simulink model "log_map_tl"  (Simulink 6.4)
settings: Solver=FixedStepDiscrete  StartTime=0.0  StopTime=50.0  FixedStep=0.1  RelTol=1e-3
PreLoadFcn:
  | if exist('tl_preloadfcn','file'), tl_preloadfcn(gcs,95); end
PostLoadFcn:
  | if exist('tl_postloadfcn','file'), tl_postloadfcn(gcs,95); end
InitFcn:
  | if exist('tlds_start','file'), tlds_start(gcs); end
undefined symbols (not defined in the file or in its folder): built, constant, Constant, Gain, in, lambda, Product, Saturate, Sum, UnitDelay, y1_0, y2_0
libraries: tllib x33
PreSaveFcn:
  | if exist('tl_presavefcn','file'), tl_presavefcn(gcs); end
settings Model: LastModifiedBy=alexh  DS_PROJECTFILE=log_map_tl.dd  TL_MAIN_DATA=struct('maxnumsimulations',10,'codeopt',struct('inliningthreshold',6,'target',['Generic ANSI-C'],'assembler',0,'optlevel',2,'linebreaklimit',100,'stateactcodinglimit',5,'functionsfor64bitops',1,'sections',1,'sfbitfields',1,'globalbitfields',0,'sharefunctions',0,'noinitstozero',0,'limidentlength',1,'decimals',1,'separatesearch',0,'cleancode',0,'optimizedbooltype',1,'keepsaturation',0,'extvarsharing',0,'outputstylefile','cconfig.xml','rootstylesheet','TL_CSourceCodeSS.xsl','addchecksum',0,'modelsaving',2,'browsecodegen',0),'frameopt',struct('exectime',1,'stacksize',1,'simconfig',['default EVM'],'targettimeout',1,'mexargs','','tcargs',''),'logopt',struct('plotinterval',0.1,'globalloggingmode',1),'export',struct('directory','.\export','sysfiles',1,'docfiles',0,'tools',0),'asapscript','asap2_all_in_one','docscript','tldoc_default','date',733152.55044912035,'codecoveragelevel',0,'rtos',struct('enablemultirate',0,'currentrtos',['generic RTOS'],'autopriority',0,'autoinitalarm',1,'alarminitwithrestart',1,'alarmactivationkind',1,'alarmstartoffset',0))  TL_MODEL_COMMENT=Type in your documentation HERE
settings DataIOCC: LimitDataPoints=off  SaveOutput=off  SaveTime=off
settings OptimizationCC: BooleanDataType=off
settings DebuggingCC: SolverPrmCheckMsg=none  StrictBusMsg=None
settings HardwareCC: TargetUnknown=on
settings GRTTargetCC: ModelReferenceCompliant=off  MatFileLogging=off

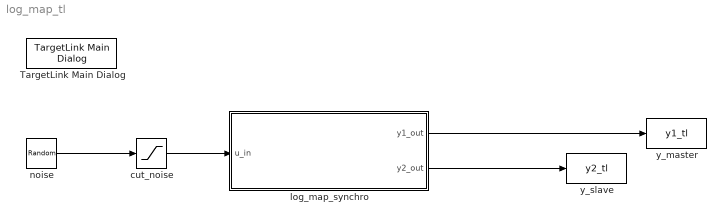
== system log_map_tl ==
  TargetLink Main Dialog : tllib/TargetLink Main Dialog  SystemSampleTime=-1  flp_block=none
  cut_noise : Saturate  UpperLimit=1  LowerLimit=0
  log_map_synchro : Subsystem  Tag=TargetLink Simulation Frame
      settings: CopyFcn=if exist('tl_copyfcn','file'), tl_copyfcn(gcbh); end  NameChangeFcn=if exist('tl_framenamechangefcn','file'), tl_framenamechangefcn(gcbh); end  OpenFcn=if exist('open_tlsubsystem','file'), open_tlsubsystem(gcbh); end
      mask Type: TL_SimFrame
      mask Display: disp('TargetLink\nModel-\nin-the-loop\nmode')
  noise : RandomNumber  Mean=0.5  SampleTime=0
  y_master : ToWorkspace  VariableName=y1_tl  SampleTime=-1  SaveFormat=Array
  y_slave : ToWorkspace  VariableName=y2_tl  SampleTime=-1  SaveFormat=Array
  wires:
  noise/1 -> cut_noise/1
  log_map_synchro/1(y1_out) -> y_master/1
  cut_noise/1 -> log_map_synchro/1(u_in)
  log_map_synchro/2(y2_out) -> y_slave/1

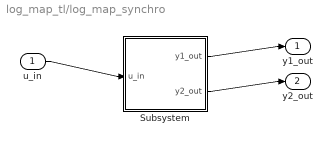
== system log_map_tl/log_map_synchro ==
  u_in : Inport  PortDimensions=1  SampleTime=0.1
      settings: NameChangeFcn=tl_check_ports(gcbh);
  Subsystem : Subsystem  Tag=struct('sfcnName','log_map_synchro_sf','subFunction','','srcSubsystem','')
      settings: OpenFcn=warndlg(get_param(gcb,'MaskHelp'),'Serious Warning');
      mask Type: TL_Enable
      mask Help: This subsystem keeps the TargetLink subsystem (subsystem with TargetLink blocks for production code generation), and is needed for the TargetLink simulation frame to work properly. DO NOT DELETE OR MODIFY IT!
  y1_out : Outport
  y2_out : Outport  Port=2
      settings: NameChangeFcn=tl_check_ports(gcbh);
  wires:
  u_in/1 -> Subsystem/1(u_in)
  Subsystem/1(y1_out) -> y1_out/1
  Subsystem/2(y2_out) -> y2_out/1

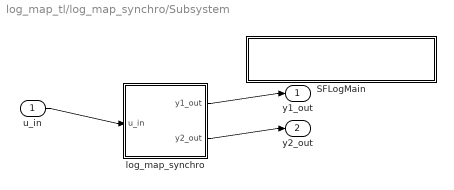
== system log_map_tl/log_map_synchro/Subsystem ==
  u_in : Inport  PortDimensions=1  SampleTime=0.1
      settings: NameChangeFcn=tl_check_ports(gcbh);
  SFLogMain : Subsystem
      mask Type: TL_StateflowLoggingMain
      mask Display:
      | plot([0 0 1 1 0 0 1 1 0],[0 1 1 0 0 0.05 0.05 0.95 0.95]);
      | disp('Stateflow Logging Main\nDO NOT DELETE')
  log_map_synchro : Subsystem  Tag=MIL Subsystem  Description=b
      settings: CopyFcn=if exist('tl_copyfcn','file'), tl_copyfcn(gcbh); end  NameChangeFcn=if exist('tl_namechangefcn','file'), tl_namechangefcn(gcbh); end  DestroyFcn=if exist('update_tl_main_dlg','file'), update_tl_main_dlg('TL_subs_display'); end
  y1_out : Outport
  y2_out : Outport  Port=2
      settings: NameChangeFcn=tl_check_ports(gcbh);
  wires:
  u_in/1 -> log_map_synchro/1(u_in)
  log_map_synchro/1(y1_out) -> y1_out/1
  log_map_synchro/2(y2_out) -> y2_out/1

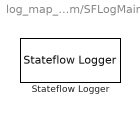
== system log_map_tl/log_map_synchro/Subsystem/SFLogMain ==
  Stateflow Logger : tllib/Extras/Stateflow Logger  data=struct('date',730486)  sflogparam=struct('charts',[],'sfblocks',[],'machines',[],'globallogopt',1,'modelname','log_map_tl','debugmodeactive',0)  flp_block=tldummylib/Stateflow Logger

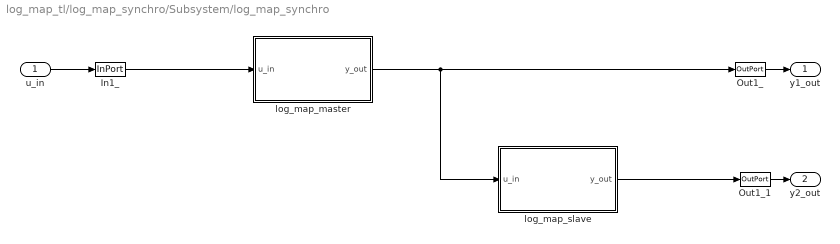
== system log_map_tl/log_map_synchro/Subsystem/log_map_synchro ==
  u_in : Inport  PortDimensions=1  SampleTime=0.1
      settings: CopyFcn=if exist('tl_check_ports','file'), tl_check_ports(gcbh); end  NameChangeFcn=if exist('tl_check_ports','file'), tl_check_ports(gcbh); end
  In1_ : tllib/InPort  SystemSampleTime=-1  data=struct('logdata',struct('maxnumvals',inf,'plotchannels',[],'loggingmode',3,'channels',1),'output',struct('width',1,'name','$S_$B','unit','','type','UInt16','offset',0,'max',1,'min',0,'freeze',1,'lsb',2^-15,'arb',0,'class','default','address','','description','','autoscalingmode',1,'lowerheadroom',1,'upperheadroom',1,'headroomunit','bit','show',0,'variable','','scaling','','keepdatatype',1,'castoutput',0),'date',733012.597276273,'message',struct('name','','component','','accessor',''),'virtual',1,'scalingvalid',0)  flp_block=none  help=|
      | InPort block of dSPACE TargetLink.
      | 
      | Input signal is read from an external variable and scaled:
      | 
      |         y = lsb * u + offset
  Out1_ : tllib/OutPort  SystemSampleTime=-1  data=struct('comment',struct('text','','placement',1),'logdata',struct('maxnumvals',inf,'plotchannels',[],'loggingmode',3,'channels',1),'output',struct('width',1,'name','$S_$B','unit','','type','UInt16','offset',0,'max',1,'min',0,'freeze',1,'lsb',2^-15,'arb',0,'class','default','address','','description','','autoscalingmode',1,'lowerheadroom',1,'upperheadroom',1,'headroomunit','bit','checkmin',0,'checkmax',0,'show',0,'variable','','scaling','','keepdatatype',1,'castoutput',0),'date',733012.597276632,'message',struct('name','','component',''),'virtual',1,'scalingvalid',0)  flp_block=none  help=|
      | OutPort block of dSPACE TargetLink.
      | 
      | Input signal is scaled:
      | 
      |         y = lsb * u + offset
  Out1_1 : tllib/OutPort  SystemSampleTime=-1  data=struct('comment',struct('text','','placement',1),'logdata',struct('maxnumvals',inf,'plotchannels',[],'loggingmode',3,'channels',1),'output',struct('width',1,'name','$S_$B','unit','','type','UInt16','offset',0,'max',1,'min',0,'freeze',1,'lsb',2^-15,'arb',0,'class','default','address','','description','','autoscalingmode',1,'lowerheadroom',1,'upperheadroom',1,'headroomunit','bit','checkmin',0,'checkmax',0,'show',0,'variable','','scaling','','keepdatatype',1,'castoutput',0),'date',733012.597276991,'message',struct('name','','component',''),'virtual',1,'scalingvalid',0)  flp_block=none  help=|
      | OutPort block of dSPACE TargetLink.
      | 
      | Input signal is scaled:
      | 
      |         y = lsb * u + offset
  log_map_master : Subsystem  TreatAsAtomicUnit=on
  log_map_slave : Subsystem  TreatAsAtomicUnit=on
  y1_out : Outport
      settings: CopyFcn=if exist('tl_check_ports','file'), tl_check_ports(gcbh); end  NameChangeFcn=if exist('tl_check_ports','file'), tl_check_ports(gcbh); end
  y2_out : Outport  Port=2
      settings: CopyFcn=if exist('tl_check_ports','file'), tl_check_ports(gcbh); end  NameChangeFcn=if exist('tl_check_ports','file'), tl_check_ports(gcbh); end
  wires:
  log_map_master/1(y_out) -> Out1_/1, log_map_slave/1(u_in)
  u_in/1 -> In1_/1
  In1_/1 -> log_map_master/1(u_in)
  Out1_/1 -> y1_out/1
  Out1_1/1 -> y2_out/1
  log_map_slave/1(y_out) -> Out1_1/1

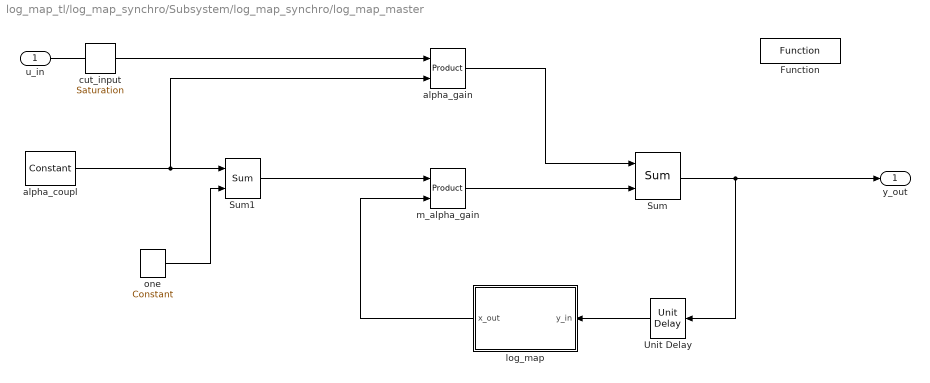
== system log_map_tl/log_map_synchro/Subsystem/log_map_synchro/log_map_master ==
  u_in : Inport
  Function : tllib/Function  SystemSampleTime=-1  data=struct('revisionNumber',9,'description','','stepfunctionname','$S_$B','stepfunctionclass','default','restartfunctionname','RESTART_$S_$B','restartfunctionclass','default','forcerestartfunction',0,'initfunctionname','INIT_$S_$B','initfunctionclass','default','forceinitfunction',0,'termfunctionname','TERM_$S_$B','termfunctionclass','default','forcetermfunction',0,'subsystemid','default','forcereuse',0,'codefile','','linkfile',0,'functionarglist',{{}},'unscaledarguments',0,'scalingpropagation',{{}},'incrcodegen',0,'ownedmodules',{{}},'simmode',1,'addtestframe',0,'destination','','codecoveragelevel',0,'codecomment','')  flp_block=none  help=|
      | Function block of dSPACE TargetLink.
      | 
      | Copy this block into a subsystem if you want separate code to be generated for it.
  Sum : tllib/Sum  data=struct('comment',struct('text','','placement',1),'logdata',struct('maxnumvals',inf,'plotchannels',[],'loggingmode',3,'channels',1),'output',struct('width',1,'name','$S_$B','unit','','type','UInt16','offset',0,'max',1,'min',0,'freeze',1,'lsb',2^-15,'arb',0,'class','default','address','','description','','autoscalingmode',1,'lowerheadroom',1,'upperheadroom',1,'headroomunit','bit','checkmin',0,'checkmax',0,'show',0,'variable','','scaling','','keepdatatype',1,'castoutput',0),'inputs','++','date',733012.597277361,'scalingvalid',0)  lower_limit=1  upper_limit=-1  flp_block=built-in/Sum  help=|
      | Sum block of dSPACE TargetLink.
      | 
      | Output signal is equal to the sum of the input signals.
      | The list of signs is specified according to conventions for Simulink Sum blocks.
  Sum1 : tllib/Sum  data=struct('comment',struct('text','','placement',1),'logdata',struct('maxnumvals',inf,'plotchannels',[],'loggingmode',3,'channels',1),'output',struct('width',1,'name','$S_$B','unit','','type','UInt16','offset',0,'max',1,'min',NaN,'freeze',1,'lsb',2^-15,'arb',0,'class','default','address','','description','','autoscalingmode',1,'lowerheadroom',1,'upperheadroom',1,'headroomunit','bit','checkmin',0,'checkmax',0,'show',0,'variable','','scaling','','keepdatatype',1,'castoutput',0),'inputs','-+','date',733012.59727772,'scalingvalid',0)  lower_limit=1  upper_limit=-1  flp_block=built-in/Sum  help=|
      | Sum block of dSPACE TargetLink.
      | 
      | Output signal is equal to the sum of the input signals.
      | The list of signs is specified according to conventions for Simulink Sum blocks.
  Unit Delay : tllib/Unit Delay  Orientation=left  SystemSampleTime=-1  data=struct('comment',struct('text','','placement',1),'logdata',struct('maxnumvals',inf,'plotchannels',[],'loggingmode',3,'channels',1),'output',struct('width',1,'name','$S_$B','unit','','type','UInt16','offset',0,'max',1,'min',0,'freeze',1,'lsb',2^-15,'arb',0,'class','default','address','','description','','autoscalingmode',1,'lowerheadroom',1,'upperheadroom',1,'headroomunit','bit','checkmin',0,'checkmax',0,'show',0,'variable','','scaling','','keepdatatype',1,'castoutput',0),'state',struct('initial','y1_0','width',1,'variable','','description','','name','X_$S_$B','address','','max',1,'min',0,'class','default','type','UInt16','scaling','','lsb',2^-15,'offset',0,'arb',0,'freeze',1,'unit',''),'dt','-1','date',733012.597278079,'scalingvalid',0)  dt=-1  X0=y1_0  flp_block=built-in/UnitDelay  help=|
      | Unit Delay block of dSPACE TargetLink.
      | 
      | Output signal is equal to the input signal of the last sample step:
      | 
      |         y(k) = u(k-1).
      | 
      | In the 1st sampling step, the output signal is initialized with 'initial condition':
      | 
      |         y(0) = initial condition
  alpha_coupl : tllib/Constant  Value=constant  OutDataType=sfix(16)  ConRadixGroup=Use specified scaling  OutScaling=2^0  data=struct('comment',struct('text','','placement',1),'output',struct('width',1,'name','$S_$B','unit','','type','UInt16','offset',0,'max',1,'min',0,'freeze',1,'lsb',2^-15,'arb',0,'class','CAL','address','','description','','value','alpha','tolerance',1,'show',0,'variable','','scaling','','keepdatatype',1),'date',733012.597278437,'dt','inf','scalingvalid',0)  constant=alpha  dt=inf  flp_block=built-in/Constant  help=|
      | Constant block of dSPACE TargetLink.
      | 
      | Output signal keeps the given constant value.
  alpha_gain : tllib/Product  data=struct('comment',struct('text','','placement',1),'logdata',struct('maxnumvals',inf,'plotchannels',[],'loggingmode',3,'channels',1),'output',struct('width',1,'name','$S_$B','unit','','type','UInt16','offset',0,'max',1,'min',0,'freeze',1,'lsb',2^-15,'arb',0,'class','default','address','','description','','autoscalingmode',1,'lowerheadroom',1,'upperheadroom',1,'headroomunit','bit','checkmin',0,'checkmax',0,'show',0,'variable','','scaling','','keepdatatype',1,'castoutput',0),'inputs','**','exceptionhandling',1,'date',733012.597278808,'scalingvalid',0)  lower_limit=1  upper_limit=-1  flp_block=built-in/Product  help=|
      | Product block of dSPACE TargetLink.
      | 
      | Output signal is equal to the product of the input signals. The input ports are specified according to conventions for Simulink Product blocks.
  cut_input : tllib/Saturation  data=struct('comment',struct('text','','placement',1),'logdata',struct('maxnumvals',inf,'plotchannels',[],'loggingmode',3,'channels',1),'output',struct('width',1,'name','$S_$B','unit','','type','UInt16','offset',0,'max',1,'min',0,'freeze',1,'lsb',2^-15,'arb',0,'class','default','address','','description','','autoscalingmode',1,'lowerheadroom',1,'upperheadroom',1,'headroomunit','bit','show',0,'variable','','scaling','','keepdatatype',1,'castoutput',0),'lowerlimit',struct('width',1,'name','$S_$B_lower','unit','','type','UInt16','offset',0,'max',NaN,'min',NaN,'freeze',1,'lsb',2^-15,'arb',0,'class','GLOBAL','address','','description','','value','0','scalar',0,'variable','','scaling','','keepdatatype',1),'upperlimit',struct('width',1,'name','$S_$B_upper','unit','','type','UInt16','offset',0,'max',NaN,'min',NaN,'freeze',1,'lsb',2^-15,'arb',0,'class','GLOBAL','address','','description','','value','1','scalar',0,'variable','','scaling','','keepdatatype',1),'date',733012.59727934,'scalingvalid',0)  lower_limit=0  upper_limit=1  flp_block=built-in/Saturate  help=|
      | Saturation block of dSPACE TargetLink.
      | 
      | The Saturation block saturates its input to the given upper and lower limit.
  log_map : Subsystem  Orientation=left  TreatAsAtomicUnit=on
  m_alpha_gain : tllib/Product  data=struct('comment',struct('text','','placement',1),'logdata',struct('maxnumvals',inf,'plotchannels',[],'loggingmode',3,'channels',1),'output',struct('width',1,'name','$S_$B','unit','','type','UInt16','offset',0,'max',1,'min',0,'freeze',1,'lsb',2^-15,'arb',0,'class','default','address','','description','','autoscalingmode',1,'lowerheadroom',1,'upperheadroom',1,'headroomunit','bit','checkmin',0,'checkmax',0,'show',0,'variable','','scaling','','keepdatatype',1,'castoutput',0),'inputs','**','exceptionhandling',1,'date',733012.597280972,'scalingvalid',0)  lower_limit=1  upper_limit=-1  flp_block=built-in/Product  help=|
      | Product block of dSPACE TargetLink.
      | 
      | Output signal is equal to the product of the input signals. The input ports are specified according to conventions for Simulink Product blocks.
  one : tllib/Constant  Value=constant  OutDataType=sfix(16)  ConRadixGroup=Use specified scaling  OutScaling=2^0  data=struct('comment',struct('text','','placement',1),'output',struct('width',1,'name','$S_$B','unit','','type','UInt16','offset',0,'max',NaN,'min',NaN,'freeze',1,'lsb',2^-15,'arb',0,'class','CONST','address','','description','','value','1','tolerance',0.001,'show',0,'variable','','scaling','','keepdatatype',1),'date',733012.597281331,'dt','inf','scalingvalid',0)  constant=1  dt=inf  flp_block=built-in/Constant  help=|
      | Constant block of dSPACE TargetLink.
      | 
      | Output signal keeps the given constant value.
  y_out : Outport
  wires:
  cut_input/1 -> alpha_gain/1
  m_alpha_gain/1 -> Sum/2
  alpha_gain/1 -> Sum/1
  log_map/1(x_out) -> m_alpha_gain/2
  Sum/1 -> y_out/1, Unit Delay/1
  u_in/1 -> cut_input/1
  Unit Delay/1 -> log_map/1(y_in)
  one/1 -> Sum1/2
  Sum1/1 -> m_alpha_gain/1
  alpha_coupl/1 -> Sum1/1, alpha_gain/2

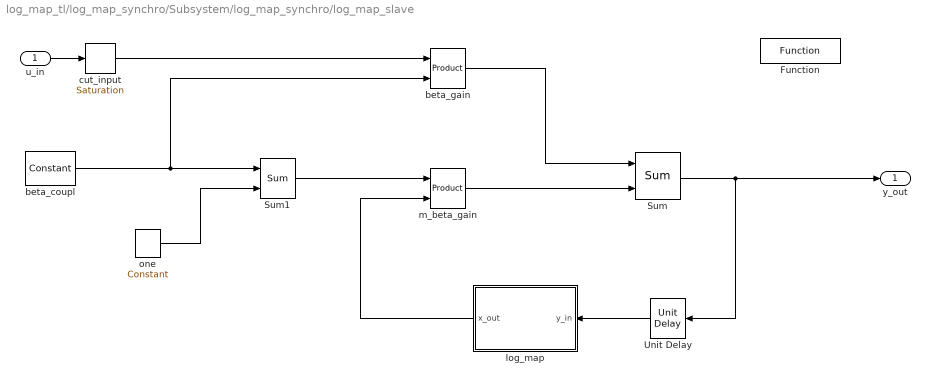
== system log_map_tl/log_map_synchro/Subsystem/log_map_synchro/log_map_slave ==
  u_in : Inport
  Function : tllib/Function  SystemSampleTime=-1  data=struct('revisionNumber',9,'description','','stepfunctionname','$S_$B','stepfunctionclass','default','restartfunctionname','RESTART_$S_$B','restartfunctionclass','default','forcerestartfunction',0,'initfunctionname','INIT_$S_$B','initfunctionclass','default','forceinitfunction',0,'termfunctionname','TERM_$S_$B','termfunctionclass','default','forcetermfunction',0,'subsystemid','default','forcereuse',0,'codefile','','linkfile',0,'functionarglist',{{}},'unscaledarguments',0,'scalingpropagation',{{}},'incrcodegen',0,'ownedmodules',{{}},'simmode',1,'addtestframe',0,'destination','','codecoveragelevel',0,'codecomment','')  flp_block=none  help=|
      | Function block of dSPACE TargetLink.
      | 
      | Copy this block into a subsystem if you want separate code to be generated for it.
  Sum : tllib/Sum  data=struct('comment',struct('text','','placement',1),'logdata',struct('maxnumvals',inf,'plotchannels',[],'loggingmode',3,'channels',1),'output',struct('width',1,'name','$S_$B','unit','','type','UInt16','offset',0,'max',1,'min',0,'freeze',1,'lsb',2^-15,'arb',0,'class','default','address','','description','','autoscalingmode',1,'lowerheadroom',1,'upperheadroom',1,'headroomunit','bit','checkmin',0,'checkmax',0,'show',0,'variable','','scaling','','keepdatatype',1,'castoutput',0),'inputs','++','date',733012.597281516,'scalingvalid',0)  lower_limit=1  upper_limit=-1  flp_block=built-in/Sum  help=|
      | Sum block of dSPACE TargetLink.
      | 
      | Output signal is equal to the sum of the input signals.
      | The list of signs is specified according to conventions for Simulink Sum blocks.
  Sum1 : tllib/Sum  data=struct('comment',struct('text','','placement',1),'logdata',struct('maxnumvals',inf,'plotchannels',[],'loggingmode',3,'channels',1),'output',struct('width',1,'name','$S_$B','unit','','type','UInt16','offset',0,'max',1,'min',NaN,'freeze',1,'lsb',2^-15,'arb',0,'class','default','address','','description','','autoscalingmode',1,'lowerheadroom',1,'upperheadroom',1,'headroomunit','bit','checkmin',0,'checkmax',0,'show',0,'variable','','scaling','','keepdatatype',1,'castoutput',0),'inputs','-+','date',733012.597281875,'scalingvalid',0)  lower_limit=1  upper_limit=-1  flp_block=built-in/Sum  help=|
      | Sum block of dSPACE TargetLink.
      | 
      | Output signal is equal to the sum of the input signals.
      | The list of signs is specified according to conventions for Simulink Sum blocks.
  Unit Delay : tllib/Unit Delay  Orientation=left  SystemSampleTime=-1  data=struct('comment',struct('text','','placement',1),'logdata',struct('maxnumvals',inf,'plotchannels',[],'loggingmode',3,'channels',1),'output',struct('width',1,'name','$S_$B','unit','','type','UInt16','offset',0,'max',1,'min',0,'freeze',1,'lsb',2^-15,'arb',0,'class','default','address','','description','','autoscalingmode',1,'lowerheadroom',1,'upperheadroom',1,'headroomunit','bit','checkmin',0,'checkmax',0,'show',0,'variable','','scaling','','keepdatatype',1,'castoutput',0),'state',struct('initial','y2_0','width',1,'variable','','description','','name','X_$S_$B','address','','max',1,'min',0,'class','default','type','UInt16','scaling','','lsb',2^-15,'offset',0,'arb',0,'freeze',1,'unit',''),'dt','-1','date',733012.597282419,'scalingvalid',0)  dt=-1  X0=y2_0  flp_block=built-in/UnitDelay  help=|
      | Unit Delay block of dSPACE TargetLink.
      | 
      | Output signal is equal to the input signal of the last sample step:
      | 
      |         y(k) = u(k-1).
      | 
      | In the 1st sampling step, the output signal is initialized with 'initial condition':
      | 
      |         y(0) = initial condition
  beta_coupl : tllib/Constant  Value=constant  OutDataType=sfix(16)  ConRadixGroup=Use specified scaling  OutScaling=2^0  data=struct('comment',struct('text','','placement',1),'output',struct('width',1,'name','$S_$B','unit','','type','UInt16','offset',0,'max',1,'min',0,'freeze',1,'lsb',2^-15,'arb',0,'class','CAL','address','','description','','value','beta','tolerance',1,'show',0,'variable','','scaling','','keepdatatype',1),'date',733012.597282778,'dt','inf','scalingvalid',0)  constant=beta  dt=inf  flp_block=built-in/Constant  help=|
      | Constant block of dSPACE TargetLink.
      | 
      | Output signal keeps the given constant value.
  beta_gain : tllib/Product  data=struct('comment',struct('text','','placement',1),'logdata',struct('maxnumvals',inf,'plotchannels',[],'loggingmode',3,'channels',1),'output',struct('width',1,'name','$S_$B','unit','','type','UInt16','offset',0,'max',1,'min',0,'freeze',1,'lsb',2^-15,'arb',0,'class','default','address','','description','','autoscalingmode',1,'lowerheadroom',1,'upperheadroom',1,'headroomunit','bit','checkmin',0,'checkmax',0,'show',0,'variable','','scaling','','keepdatatype',1,'castoutput',0),'inputs','**','exceptionhandling',1,'date',733012.597282963,'scalingvalid',0)  lower_limit=1  upper_limit=-1  flp_block=built-in/Product  help=|
      | Product block of dSPACE TargetLink.
      | 
      | Output signal is equal to the product of the input signals. The input ports are specified according to conventions for Simulink Product blocks.
  cut_input : tllib/Saturation  data=struct('comment',struct('text','','placement',1),'logdata',struct('maxnumvals',inf,'plotchannels',[],'loggingmode',3,'channels',1),'output',struct('width',1,'name','$S_$B','unit','','type','UInt16','offset',0,'max',1,'min',0,'freeze',1,'lsb',2^-15,'arb',0,'class','default','address','','description','','autoscalingmode',1,'lowerheadroom',1,'upperheadroom',1,'headroomunit','bit','show',0,'variable','','scaling','','keepdatatype',1,'castoutput',0),'lowerlimit',struct('width',1,'name','$S_$B_lower','unit','','type','UInt16','offset',0,'max',NaN,'min',NaN,'freeze',1,'lsb',2^-15,'arb',0,'class','GLOBAL','address','','description','','value','0','scalar',0,'variable','','scaling','','keepdatatype',1),'upperlimit',struct('width',1,'name','$S_$B_upper','unit','','type','UInt16','offset',0,'max',NaN,'min',NaN,'freeze',1,'lsb',2^-15,'arb',0,'class','GLOBAL','address','','description','','value','1','scalar',0,'variable','','scaling','','keepdatatype',1),'date',733012.597283681,'scalingvalid',0)  lower_limit=0  upper_limit=1  flp_block=built-in/Saturate  help=|
      | Saturation block of dSPACE TargetLink.
      | 
      | The Saturation block saturates its input to the given upper and lower limit.
  log_map : Subsystem  Orientation=left  TreatAsAtomicUnit=on
  m_beta_gain : tllib/Product  data=struct('comment',struct('text','','placement',1),'logdata',struct('maxnumvals',inf,'plotchannels',[],'loggingmode',3,'channels',1),'output',struct('width',1,'name','$S_$B','unit','','type','UInt16','offset',0,'max',1,'min',0,'freeze',1,'lsb',2^-15,'arb',0,'class','default','address','','description','','autoscalingmode',1,'lowerheadroom',1,'upperheadroom',1,'headroomunit','bit','checkmin',0,'checkmax',0,'show',0,'variable','','scaling','','keepdatatype',1,'castoutput',0),'inputs','**','exceptionhandling',1,'date',733012.597285312,'scalingvalid',0)  lower_limit=1  upper_limit=-1  flp_block=built-in/Product  help=|
      | Product block of dSPACE TargetLink.
      | 
      | Output signal is equal to the product of the input signals. The input ports are specified according to conventions for Simulink Product blocks.
  one : tllib/Constant  Value=constant  OutDataType=sfix(16)  ConRadixGroup=Use specified scaling  OutScaling=2^0  data=struct('comment',struct('text','','placement',1),'output',struct('width',1,'name','$S_$B','unit','','type','UInt16','offset',0,'max',NaN,'min',NaN,'freeze',1,'lsb',2^-15,'arb',0,'class','CONST','address','','description','','value','1','tolerance',0.001,'show',0,'variable','','scaling','','keepdatatype',1),'date',733012.597285486,'dt','inf','scalingvalid',0)  constant=1  dt=inf  flp_block=built-in/Constant  help=|
      | Constant block of dSPACE TargetLink.
      | 
      | Output signal keeps the given constant value.
  y_out : Outport
  wires:
  Unit Delay/1 -> log_map/1(y_in)
  u_in/1 -> cut_input/1
  Sum/1 -> Unit Delay/1, y_out/1
  log_map/1(x_out) -> m_beta_gain/2
  beta_gain/1 -> Sum/1
  m_beta_gain/1 -> Sum/2
  cut_input/1 -> beta_gain/1
  Sum1/1 -> m_beta_gain/1
  beta_coupl/1 -> Sum1/1, beta_gain/2
  one/1 -> Sum1/2

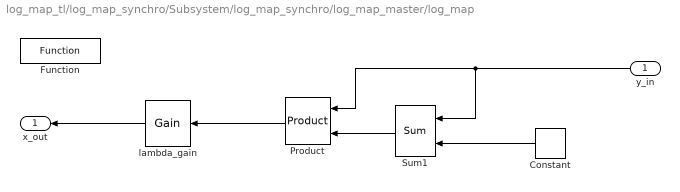
== system log_map_tl/log_map_synchro/Subsystem/log_map_synchro/log_map_master/log_map ==
  y_in : Inport  Orientation=left
  Constant : tllib/Constant  Orientation=left  Value=constant  OutDataType=sfix(16)  ConRadixGroup=Use specified scaling  OutScaling=2^0  data=struct('comment',struct('text','','placement',1),'output',struct('width',1,'name','$S_$B','unit','','type','UInt16','offset',0,'max',NaN,'min',NaN,'freeze',1,'lsb',2^-15,'arb',0,'class','CONST','address','','description','','value','1','tolerance',1,'show',0,'variable','','scaling','','keepdatatype',1),'date',733012.597279525,'dt','inf','scalingvalid',0)  constant=1  dt=inf  flp_block=built-in/Constant  help=|
      | Constant block of dSPACE TargetLink.
      | 
      | Output signal keeps the given constant value.
  Function : tllib/Function  SystemSampleTime=-1  data=struct('revisionNumber',9,'description','','stepfunctionname','$S_$B','stepfunctionclass','default','restartfunctionname','RESTART_$S_$B','restartfunctionclass','default','forcerestartfunction',0,'initfunctionname','INIT_$S_$B','initfunctionclass','default','forceinitfunction',0,'termfunctionname','TERM_$S_$B','termfunctionclass','default','forcetermfunction',0,'subsystemid','default','forcereuse',0,'codefile','','linkfile',0,'functionarglist',{{}},'unscaledarguments',0,'scalingpropagation',{{}},'incrcodegen',0,'ownedmodules',{{}},'simmode',1,'addtestframe',0,'destination','','codecoveragelevel',0,'codecomment','')  flp_block=none  help=|
      | Function block of dSPACE TargetLink.
      | 
      | Copy this block into a subsystem if you want separate code to be generated for it.
  Product : tllib/Product  Orientation=left  data=struct('comment',struct('text','','placement',1),'logdata',struct('maxnumvals',inf,'plotchannels',[],'loggingmode',3,'channels',1),'output',struct('width',1,'name','$S_$B','unit','','type','UInt16','offset',0,'max',1,'min',0,'freeze',1,'lsb',2^-15,'arb',0,'class','default','address','','description','','autoscalingmode',1,'lowerheadroom',1,'upperheadroom',1,'headroomunit','bit','checkmin',0,'checkmax',0,'show',0,'variable','','scaling','','keepdatatype',1,'castoutput',0),'inputs','2','exceptionhandling',1,'date',733012.597279884,'scalingvalid',0)  lower_limit=1  upper_limit=-1  flp_block=built-in/Product  help=|
      | Product block of dSPACE TargetLink.
      | 
      | Output signal is equal to the product of the input signals. The input ports are specified according to conventions for Simulink Product blocks.
  Sum1 : tllib/Sum  Orientation=left  data=struct('comment',struct('text','','placement',1),'logdata',struct('maxnumvals',inf,'plotchannels',[],'loggingmode',3,'channels',1),'output',struct('width',1,'name','$S_$B','unit','','type','UInt16','offset',0,'max',1,'min',0,'freeze',1,'lsb',2^-15,'arb',0,'class','default','address','','description','','autoscalingmode',1,'lowerheadroom',1,'upperheadroom',1,'headroomunit','bit','checkmin',0,'checkmax',0,'show',0,'variable','','scaling','','keepdatatype',1,'castoutput',0),'inputs','-+','date',733012.597280243,'scalingvalid',0)  lower_limit=1  upper_limit=-1  flp_block=built-in/Sum  help=|
      | Sum block of dSPACE TargetLink.
      | 
      | Output signal is equal to the sum of the input signals.
      | The list of signs is specified according to conventions for Simulink Sum blocks.
  lambda_gain : tllib/Gain  Orientation=left  SystemSampleTime=-1  data=struct('comment',struct('text','','placement',1),'logdata',struct('maxnumvals',inf,'plotchannels',[],'loggingmode',3,'channels',1),'output',struct('width',1,'name','$S_$B','unit','','type','UInt16','offset',0,'max',1,'min',0,'freeze',1,'lsb',2^-15,'arb',0,'class','default','address','','description','','autoscalingmode',1,'lowerheadroom',1,'upperheadroom',1,'headroomunit','bit','checkmin',0,'checkmax',0,'show',0,'variable','','scaling','','keepdatatype',1,'castoutput',0),'gain',struct('width',1,'name','$S_$B_gain','unit','','type','Int16','offset',0,'max',4,'min',0,'freeze',1,'lsb',2^-12,'arb',0,'class','CAL','address','','description','','value','lambda','scalar',0,'tolerance',1,'variable','','scaling','','keepdatatype',1),'date',733012.597280613,'scalingvalid',0)  gain=lambda  flp_block=built-in/Gain  help=|
      | Gain block of dSPACE TargetLink.
      | 
      | Output signal is equal to the product of the input signal and the gain value:
      |         y = G u
  x_out : Outport  Orientation=left
  wires:
  Constant/1 -> Sum1/2
  Sum1/1 -> Product/2
  y_in/1 -> Sum1/1, Product/1
  Product/1 -> lambda_gain/1
  lambda_gain/1 -> x_out/1

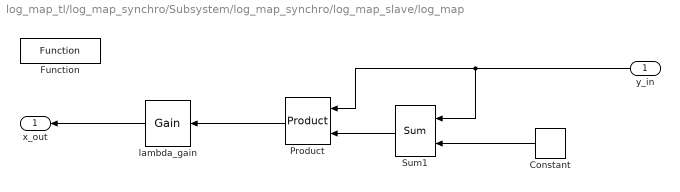
== system log_map_tl/log_map_synchro/Subsystem/log_map_synchro/log_map_slave/log_map ==
  y_in : Inport  Orientation=left
  Constant : tllib/Constant  Orientation=left  Value=constant  OutDataType=sfix(16)  ConRadixGroup=Use specified scaling  OutScaling=2^0  data=struct('comment',struct('text','','placement',1),'output',struct('width',1,'name','$S_$B','unit','','type','UInt16','offset',0,'max',NaN,'min',NaN,'freeze',1,'lsb',2^-15,'arb',0,'class','CONST','address','','description','','value','1','tolerance',1,'show',0,'variable','','scaling','','keepdatatype',1),'date',733012.597283866,'dt','inf','scalingvalid',0)  constant=1  dt=inf  flp_block=built-in/Constant  help=|
      | Constant block of dSPACE TargetLink.
      | 
      | Output signal keeps the given constant value.
  Function : tllib/Function  SystemSampleTime=-1  data=struct('revisionNumber',9,'description','','stepfunctionname','$S_$B','stepfunctionclass','default','restartfunctionname','RESTART_$S_$B','restartfunctionclass','default','forcerestartfunction',0,'initfunctionname','INIT_$S_$B','initfunctionclass','default','forceinitfunction',0,'termfunctionname','TERM_$S_$B','termfunctionclass','default','forcetermfunction',0,'subsystemid','default','forcereuse',0,'codefile','','linkfile',0,'functionarglist',{{}},'unscaledarguments',0,'scalingpropagation',{{}},'incrcodegen',0,'ownedmodules',{{}},'simmode',1,'addtestframe',0,'destination','','codecoveragelevel',0,'codecomment','')  flp_block=none  help=|
      | Function block of dSPACE TargetLink.
      | 
      | Copy this block into a subsystem if you want separate code to be generated for it.
  Product : tllib/Product  Orientation=left  data=struct('comment',struct('text','','placement',1),'logdata',struct('maxnumvals',inf,'plotchannels',[],'loggingmode',3,'channels',1),'output',struct('width',1,'name','$S_$B','unit','','type','UInt16','offset',0,'max',1,'min',0,'freeze',1,'lsb',2^-15,'arb',0,'class','default','address','','description','','autoscalingmode',1,'lowerheadroom',1,'upperheadroom',1,'headroomunit','bit','checkmin',0,'checkmax',0,'show',0,'variable','','scaling','','keepdatatype',1,'castoutput',0),'inputs','2','exceptionhandling',1,'date',733012.597284225,'scalingvalid',0)  lower_limit=1  upper_limit=-1  flp_block=built-in/Product  help=|
      | Product block of dSPACE TargetLink.
      | 
      | Output signal is equal to the product of the input signals. The input ports are specified according to conventions for Simulink Product blocks.
  Sum1 : tllib/Sum  Orientation=left  data=struct('comment',struct('text','','placement',1),'logdata',struct('maxnumvals',inf,'plotchannels',[],'loggingmode',3,'channels',1),'output',struct('width',1,'name','$S_$B','unit','','type','UInt16','offset',0,'max',1,'min',0,'freeze',1,'lsb',2^-15,'arb',0,'class','default','address','','description','','autoscalingmode',1,'lowerheadroom',1,'upperheadroom',1,'headroomunit','bit','checkmin',0,'checkmax',0,'show',0,'variable','','scaling','','keepdatatype',1,'castoutput',0),'inputs','-+','date',733012.597284583,'scalingvalid',0)  lower_limit=1  upper_limit=-1  flp_block=built-in/Sum  help=|
      | Sum block of dSPACE TargetLink.
      | 
      | Output signal is equal to the sum of the input signals.
      | The list of signs is specified according to conventions for Simulink Sum blocks.
  lambda_gain : tllib/Gain  Orientation=left  SystemSampleTime=-1  data=struct('comment',struct('text','','placement',1),'logdata',struct('maxnumvals',inf,'plotchannels',[],'loggingmode',3,'channels',1),'output',struct('width',1,'name','$S_$B','unit','','type','UInt16','offset',0,'max',1,'min',0,'freeze',1,'lsb',2^-15,'arb',0,'class','default','address','','description','','autoscalingmode',1,'lowerheadroom',1,'upperheadroom',1,'headroomunit','bit','checkmin',0,'checkmax',0,'show',0,'variable','','scaling','','keepdatatype',1,'castoutput',0),'gain',struct('width',1,'name','$S_$B_gain','unit','','type','Int16','offset',0,'max',4,'min',0,'freeze',1,'lsb',2^-12,'arb',0,'class','CAL','address','','description','','value','lambda','scalar',0,'tolerance',1,'variable','','scaling','','keepdatatype',1),'date',733012.597284954,'scalingvalid',0)  gain=lambda  flp_block=built-in/Gain  help=|
      | Gain block of dSPACE TargetLink.
      | 
      | Output signal is equal to the product of the input signal and the gain value:
      |         y = G u
  x_out : Outport  Orientation=left
  wires:
  lambda_gain/1 -> x_out/1
  Product/1 -> lambda_gain/1
  y_in/1 -> Product/1, Sum1/1
  Sum1/1 -> Product/2
  Constant/1 -> Sum1/2
